simulink model "Vienna_SVM"  (Simulink 7.6)
settings: Solver=ode23tb  StartTime=0.0  StopTime=1.5  RelTol=1e-3
libraries: powerlib x31, powerlib_extras x7, simulink x5
settings Model: Creator=huanglei  LastModifiedBy=huanglei

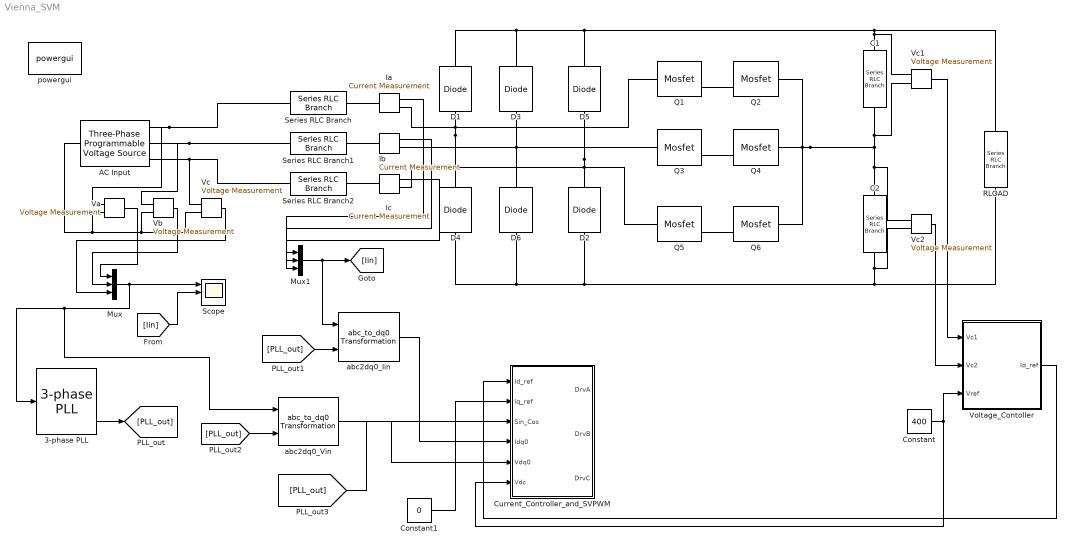
== system Vienna_SVM ==
  3-phase PLL : powerlib_extras/Control  Blocks/3-phase PLL  DialogController=POWERSYS.PowerSysDialog  SystemSampleTime=-1  Par_Init=[0 50]  ParK=[ 180 3200 1 ]  AGC=off
  AC Input : powerlib/Electrical Sources/Three-Phase Programmable Voltage Source  DialogController=POWERSYS.PowerSysDialog  SystemSampleTime=-1  PositiveSequence="[190  0 50]"  VariationEntity=None  VariationType=Step  VariationStep=0.5  VariationRate=10  VariationMagnitude=0.3  VariationFrequency=2  VariationTiming=[1 2]  VariationPhaseA=off  Amplitudes=[1 0.8 1.2 1.0]  TimeValues=[0 0.1 0.15 0.2]  HarmonicGeneration=off  HarmonicA=[3 0.2 -25 0]  HarmonicB=[2 0.15 35 2]  Timing="[0.05  3]"
  C1 : powerlib/Elements/Series RLC Branch  DialogController=POWERSYS.PowerSysDialog  PhysicalDomain=powersysdomain  SubClassName=unknown  LeftPortType=p1  RightPortType=p1  LConnTagsString=__new0  RConnTagsString=__new0  BranchType=C  Resistance=1  Inductance=1e-3  SetiL0=off  InitialCurrent=0  Capacitance=1e-3  Setx0=off  InitialVoltage=0  Measurements=None
  C2 : powerlib/Elements/Series RLC Branch  DialogController=POWERSYS.PowerSysDialog  PhysicalDomain=powersysdomain  SubClassName=unknown  LeftPortType=p1  RightPortType=p1  LConnTagsString=__new0  RConnTagsString=__new0  BranchType=C  Resistance=1  Inductance=1e-3  SetiL0=off  InitialCurrent=0  Capacitance=1e-3  Setx0=off  InitialVoltage=0  Measurements=None
  Constant : Constant  Value=400
  Constant1 : Constant  Value=0
  Current_Controller_and_SVPWM : Subsystem
  D{1..6} (6 alike) : powerlib/Power Electronics/Diode  DialogController=POWERSYS.PowerSysDialog  SystemSampleTime=-1  Ron=0.001  Lon=0  Vf=0.8  IC=0  UseSnubber=off  Rs=500  Cs=250e-9  Measurements=off
  Ia : powerlib/Measurements/Current Measurement  DialogController=POWERSYS.PowerSysDialog  SystemSampleTime=-1  PhasorSimulation=off  OutputType=Complex  PSBequivalent=0
  Ib : powerlib/Measurements/Current Measurement  DialogController=POWERSYS.PowerSysDialog  SystemSampleTime=-1  PhasorSimulation=off  OutputType=Complex  PSBequivalent=0
  Ic : powerlib/Measurements/Current Measurement  DialogController=POWERSYS.PowerSysDialog  SystemSampleTime=-1  PhasorSimulation=off  OutputType=Complex  PSBequivalent=0
  Mux : Mux  Inputs=3
  Mux1 : Mux  Inputs=3
  Q1 : powerlib/Power Electronics/Mosfet  DialogController=POWERSYS.PowerSysDialog  SystemSampleTime=-1  Ron=0.01  Lon=0  Rd=0.01  Vfd=0  IC=0  Rs=1e5  Cs=inf  Measurements=off
  Q{2..6} (5 alike) : powerlib/Power Electronics/Mosfet  DialogController=POWERSYS.PowerSysDialog  SystemSampleTime=-1  Ron=0.1  Lon=0  Rd=0.01  Vfd=0  IC=0  Rs=1e5  Cs=inf  Measurements=off
  RLOAD : powerlib/Elements/Series RLC Branch  DialogController=POWERSYS.PowerSysDialog  PhysicalDomain=powersysdomain  SubClassName=unknown  LeftPortType=p1  RightPortType=p1  LConnTagsString=__new0  RConnTagsString=__new0  BranchType=R  Resistance=80  Inductance=1e-3  SetiL0=off  InitialCurrent=0  Capacitance=1e-6  Setx0=off  InitialVoltage=0  Measurements=None
  Scope : Scope  NumInputPorts=3
      settings: YMin=-5~-5~-5  YMax=5~5~5
  Series RLC Branch : powerlib/Elements/Series RLC Branch  DialogController=POWERSYS.PowerSysDialog  PhysicalDomain=powersysdomain  SubClassName=unknown  LeftPortType=p1  RightPortType=p1  LConnTagsString=__new0  RConnTagsString=__new0  BranchType=RL  Resistance=0  Inductance=3.5e-3  SetiL0=off  InitialCurrent=0  Capacitance=1e-6  Setx0=off  InitialVoltage=0  Measurements=None
  Series RLC Branch1 : powerlib/Elements/Series RLC Branch  DialogController=POWERSYS.PowerSysDialog  PhysicalDomain=powersysdomain  SubClassName=unknown  LeftPortType=p1  RightPortType=p1  LConnTagsString=__new0  RConnTagsString=__new0  BranchType=RL  Resistance=0  Inductance=3.5e-3  SetiL0=off  InitialCurrent=0  Capacitance=1e-6  Setx0=off  InitialVoltage=0  Measurements=None
  Series RLC Branch2 : powerlib/Elements/Series RLC Branch  DialogController=POWERSYS.PowerSysDialog  PhysicalDomain=powersysdomain  SubClassName=unknown  LeftPortType=p1  RightPortType=p1  LConnTagsString=__new0  RConnTagsString=__new0  BranchType=RL  Resistance=0  Inductance=3.5e-3  SetiL0=off  InitialCurrent=0  Capacitance=1e-6  Setx0=off  InitialVoltage=0  Measurements=None
  Va : powerlib/Measurements/Voltage Measurement  DialogController=POWERSYS.PowerSysDialog  SystemSampleTime=-1  PhasorSimulation=off  OutputType=Complex  PSBequivalent=0
  Vb : powerlib/Measurements/Voltage Measurement  DialogController=POWERSYS.PowerSysDialog  SystemSampleTime=-1  PhasorSimulation=off  OutputType=Complex  PSBequivalent=0
  Vc : powerlib/Measurements/Voltage Measurement  DialogController=POWERSYS.PowerSysDialog  SystemSampleTime=-1  PhasorSimulation=off  OutputType=Complex  PSBequivalent=0
  Vc1 : powerlib/Measurements/Voltage Measurement  DialogController=POWERSYS.PowerSysDialog  SystemSampleTime=-1  PhasorSimulation=off  OutputType=Complex  PSBequivalent=0
  Vc2 : powerlib/Measurements/Voltage Measurement  DialogController=POWERSYS.PowerSysDialog  SystemSampleTime=-1  PhasorSimulation=off  OutputType=Complex  PSBequivalent=0
  Voltage_Contoller : Subsystem
  abc2dq0_Iin : powerlib_extras/Measurements/abc_to_dq0 Transformation  DialogController=POWERSYS.PowerSysDialog  SystemSampleTime=-1
  abc2dq0_Vin : powerlib_extras/Measurements/abc_to_dq0 Transformation  DialogController=POWERSYS.PowerSysDialog  SystemSampleTime=-1
  powergui : powerlib/powergui  Priority=1  SystemSampleTime=-1  SimulationMode=Discrete  SampleTime=50e-6  frequency=60  SPID=off  DisableSnubberDevices=off  DisableRonSwitches=off  DisableVfSwitches=off  SwTol=0  Interpol=off  frequencyindice=50  echomessages=off  HookPort=off  DisplayEquations=off  FunctionMessages=off  EnableUseOfTLC=off  x0status=blocks  RestoreLinks=warning  ResistiveCurrentMeasurement=off  Ylog=off  Xlog=on  ShowGrid=off  save=off  variable=ZData  ZoomFFT=off  StartTime=0.0  cycles=1  DisplayStyle=1  FreqAxis=off  MaxFrequency=1000  frequencyindicesteady=1  display=off  methode=off
  wires:
  Vb/1 -> Mux/2
  Va/1 -> Mux/1
  Vc/1 -> Mux/3
  Mux/1 -> Scope/1, 3-phase PLL/1, abc2dq0_Vin/1
  Ia/1 -> Mux1/1
  Ib/1 -> Mux1/2
  Ic/1 -> Mux1/3
  Mux1/1 -> [Iin], abc2dq0_Iin/1
  [Iin] -> Scope/2
  [PLL_out] -> abc2dq0_Iin/2
  3-phase PLL/3 -> [PLL_out]
  [PLL_out] -> abc2dq0_Vin/2
  Constant/1 -> Voltage_Contoller/3(Vref), Current_Controller_and_SVPWM/6(Vdc)
  Vc1/1 -> Voltage_Contoller/1(Vc1)
  Vc2/1 -> Voltage_Contoller/2(Vc2)
  abc2dq0_Iin/1 -> Current_Controller_and_SVPWM/4(Idq0)
  abc2dq0_Vin/1 -> Current_Controller_and_SVPWM/5(Vdq0)
  [PLL_out] -> Current_Controller_and_SVPWM/3(Sin_Cos)
  Constant1/1 -> Current_Controller_and_SVPWM/2(Iq_ref)
  Voltage_Contoller/1(Id_ref) -> Current_Controller_and_SVPWM/1(Id_ref)
  connections:
  AC Input/RConn1 -- Series RLC Branch/LConn1 -- Va/LConn1
  AC Input/RConn2 -- Series RLC Branch1/LConn1 -- Vb/LConn1
  AC Input/RConn3 -- Series RLC Branch2/LConn1 -- Vc/LConn1
  Vc/LConn2 -- Vb/LConn2 -- AC Input/LConn1 -- Va/LConn2
  Series RLC Branch/RConn1 -- Ia/LConn1
  Series RLC Branch1/RConn1 -- Ib/LConn1
  Series RLC Branch2/RConn1 -- Ic/LConn1
  Ia/RConn1 -- D1/LConn1 -- D4/RConn1 -- Q1/RConn1
  D3/LConn1 -- D6/RConn1 -- Ib/RConn1 -- Q3/RConn1
  Ic/RConn1 -- D5/LConn1 -- D2/RConn1 -- Q5/RConn1
  D1/RConn1 -- D3/RConn1 -- D5/RConn1 -- RLOAD/LConn1 -- C1/LConn1 -- Vc1/LConn1
  C2/RConn1 -- D4/LConn1 -- D6/LConn1 -- D2/LConn1 -- RLOAD/RConn1 -- Vc2/LConn2
  Q4/RConn1 -- Q2/RConn1 -- Q6/RConn1 -- C1/RConn1 -- Vc1/LConn2 -- C2/LConn1 -- Vc2/LConn1
  Q1/LConn1 -- Q2/LConn1
  Q3/LConn1 -- Q4/LConn1
  Q5/LConn1 -- Q6/LConn1

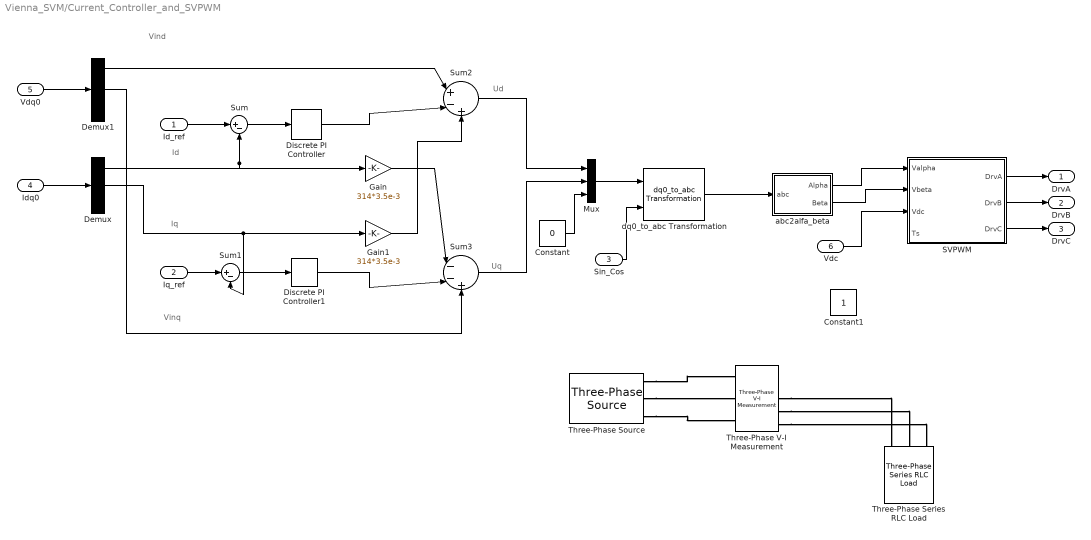
== system Vienna_SVM/Current_Controller_and_SVPWM ==
  note: Ud
  note: Uq
  note: Vind
  note: Vinq
  note: Id
  note: Iq
  Id_ref : Inport
  Iq_ref : Inport  Port=2
  Sin_Cos : Inport  Port=3
  Idq0 : Inport  Port=4
  Vdq0 : Inport  Port=5
  Vdc : Inport  Port=6
  Constant : Constant  Value=0
  Constant1 : Constant
  Demux : Demux  Outputs=3
  Demux1 : Demux  Outputs=3
  Discrete PI Controller : powerlib_extras/Discrete  Control Blocks/Discrete PI Controller  DialogController=POWERSYS.PowerSysDialog  SystemSampleTime=-1  Kp=0.1  Ki=1  Par_Limits=[1e6 -1e6]  Init=0  Ts=50e-6
  Discrete PI Controller1 : powerlib_extras/Discrete  Control Blocks/Discrete PI Controller  DialogController=POWERSYS.PowerSysDialog  SystemSampleTime=-1  Kp=0.1  Ki=1  Par_Limits=[1e6 -1e6]  Init=0  Ts=50e-6
  Gain : Gain  Gain=314*3.5e-3
  Gain1 : Gain  Gain=314*3.5e-3
  Mux : Mux  Inputs=3
  SVPWM : Subsystem
  Sum : Sum  Inputs=|+-
  Sum1 : Sum  Inputs=|+-
  Sum2 : Sum  Inputs=|+-+
  Sum3 : Sum  Inputs=|--+
  Three-Phase Series RLC Load : powerlib/Elements/Three-Phase Series RLC Load  DialogController=POWERSYS.PowerSysDialog  PhysicalDomain=powersysdomain  SubClassName=unknown  LeftPortType=p1  RightPortType=p1  LConnTagsString=A|B|C  Configuration=Y (grounded)  NominalVoltage=1000  NominalFrequency=60  ActivePower=10e3  InductivePower=100  CapacitivePower=100  Measurements=None
  Three-Phase V-I Measurement : powerlib/Measurements/Three-Phase V-I Measurement  DialogController=POWERSYS.PowerSysDialog  SystemSampleTime=-1  VoltageMeasurement=phase-to-ground  SetLabelV=off  LabelV=Vabc  Vpu=off  VpuLL=off  CurrentMeasurement=yes  SetLabelI=off  LabelI=Iabc  Ipu=off  Pbase=100e6  Vbase=500e3  OutputType=Complex  PhasorSimulation=off  PSBequivalent=0
  Three-Phase Source : powerlib/Electrical Sources/Three-Phase Source  DialogController=POWERSYS.PowerSysDialog  SystemSampleTime=-1  Voltage=381  PhaseAngle=0  Frequency=50  InternalConnection=Yn  SpecifyImpedance=on  Resistance=0.8929  Inductance=16.58e-3  ShortCircuitLevel=100e6  BaseVoltage=25e3  XRratio=7
  abc2alfa_beta : Subsystem
  dq0_to_abc Transformation : powerlib_extras/Measurements/dq0_to_abc Transformation  DialogController=POWERSYS.PowerSysDialog  SystemSampleTime=-1
  DrvA : Outport
  DrvB : Outport  Port=2
  DrvC : Outport  Port=3
  wires:
  Id_ref/1 -> Sum/1
  Demux/1 -> Sum/2, Gain/1
  Sum/1 -> Discrete PI Controller/1
  Iq_ref/1 -> Sum1/1
  Sum1/1 -> Discrete PI Controller1/1
  Discrete PI Controller1/1 -> Sum3/2
  Discrete PI Controller/1 -> Sum2/2
  Gain1/1 -> Sum2/3
  Gain/1 -> Sum3/1
  Demux1/1 -> Sum2/1
  Sum2/1 -> Mux/1
  Sum3/1 -> Mux/2
  Constant/1 -> Mux/3
  Mux/1 -> dq0_to_abc Transformation/1
  Sin_Cos/1 -> dq0_to_abc Transformation/2
  Idq0/1 -> Demux/1
  Demux/2 -> Sum1/2, Gain1/1
  Vdq0/1 -> Demux1/1
  Demux1/2 -> Sum3/3
  SVPWM/1(DrvA) -> DrvA/1
  SVPWM/2(DrvB) -> DrvB/1
  SVPWM/3(DrvC) -> DrvC/1
  abc2alfa_beta/1(Alpha) -> SVPWM/1(Valpha)
  abc2alfa_beta/2(Beta) -> SVPWM/2(Vbeta)
  dq0_to_abc Transformation/1 -> abc2alfa_beta/1(abc)
  Vdc/1 -> SVPWM/3(Vdc)
  connections:
  Three-Phase Source/RConn1 -- Three-Phase V-I Measurement/LConn1
  Three-Phase Source/RConn2 -- Three-Phase V-I Measurement/LConn2
  Three-Phase Source/RConn3 -- Three-Phase V-I Measurement/LConn3
  Three-Phase V-I Measurement/RConn3 -- Three-Phase Series RLC Load/LConn3
  Three-Phase V-I Measurement/RConn2 -- Three-Phase Series RLC Load/LConn2
  Three-Phase V-I Measurement/RConn1 -- Three-Phase Series RLC Load/LConn1

== system Vienna_SVM/Voltage_Contoller ==
  Vc1 : Inport
  Vc2 : Inport  Port=2
  Vref : Inport  Port=3
  Discrete PID Controller1 : powerlib_extras/Discrete  Control Blocks/Discrete PID Controller  DialogController=POWERSYS.PowerSysDialog  SystemSampleTime=-1  Kp=1  Ki=1  Kd=1  TcD=1  Par_Limits=[100 -100]  Init=0  Ts=0.5
  Saturation : Saturate
  Sum : Sum  Inputs=|++
  Sum1 : Sum  Inputs=|+-
  Id_ref : Outport
  wires:
  Vc1/1 -> Sum/1
  Vc2/1 -> Sum/2
  Vref/1 -> Sum1/1
  Sum/1 -> Sum1/2
  Sum1/1 -> Discrete PID Controller1/1
  Discrete PID Controller1/1 -> Saturation/1
  Saturation/1 -> Id_ref/1

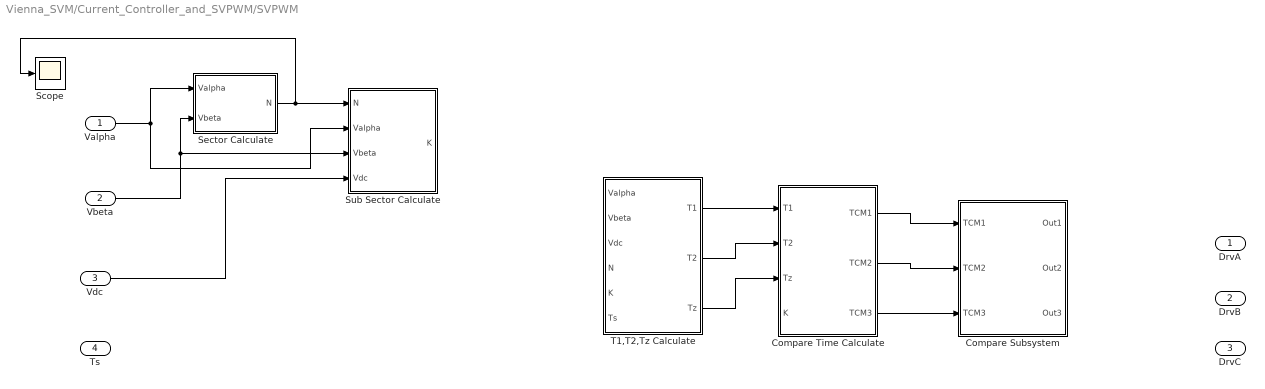
== system Vienna_SVM/Current_Controller_and_SVPWM/SVPWM ==
  Valpha : Inport
  Vbeta : Inport  Port=2
  Vdc : Inport  Port=3
  Ts : Inport  Port=4
  Compare Subsystem : Subsystem
  Compare Time Calculate : Subsystem
  Scope : Scope
  Sector Calculate : Subsystem
  Sub Sector Calculate : Subsystem
  T1,T2,Tz Calculate : Subsystem
  DrvA : Outport
  DrvB : Outport  Port=2
  DrvC : Outport  Port=3
  wires:
  Valpha/1 -> Sector Calculate/1(Valpha), Sub Sector Calculate/2(Valpha)
  Vbeta/1 -> Sector Calculate/2(Vbeta), Sub Sector Calculate/3(Vbeta)
  Sector Calculate/1(N) -> Scope/1, Sub Sector Calculate/1(N)
  Vdc/1 -> Sub Sector Calculate/4(Vdc)
  T1,T2,Tz Calculate/1(T1) -> Compare Time Calculate/1(T1)
  T1,T2,Tz Calculate/2(T2) -> Compare Time Calculate/2(T2)
  T1,T2,Tz Calculate/3(Tz) -> Compare Time Calculate/3(Tz)
  Compare Time Calculate/1(TCM1) -> Compare Subsystem/1(TCM1)
  Compare Time Calculate/3(TCM3) -> Compare Subsystem/3(TCM3)
  Compare Time Calculate/2(TCM2) -> Compare Subsystem/2(TCM2)

== system Vienna_SVM/Current_Controller_and_SVPWM/abc2alfa_beta ==
  abc : Inport
  Demux : Demux  Outputs=3
  Gain : Gain  Gain=2
  Gain1 : Gain  Gain=1/3
  Gain2 : Gain  Gain=sqrt(3)/3
  Scope : Scope  NumInputPorts=3
      settings: YMin=-5~-5~-5  YMax=5~5~5  SaveName=ScopeData2
  Sum : Sum  Inputs=|+--
  Sum2 : Sum  Inputs=|-+
  Alpha : Outport
  Beta : Outport  Port=2
  wires:
  Demux/1 -> Gain/1, Scope/1
  Gain/1 -> Sum/1
  Demux/2 -> Sum/2, Sum2/2, Scope/2
  Demux/3 -> Sum/3, Sum2/1, Scope/3
  Sum/1 -> Gain1/1
  Sum2/1 -> Gain2/1
  abc/1 -> Demux/1
  Gain1/1 -> Alpha/1
  Gain2/1 -> Beta/1

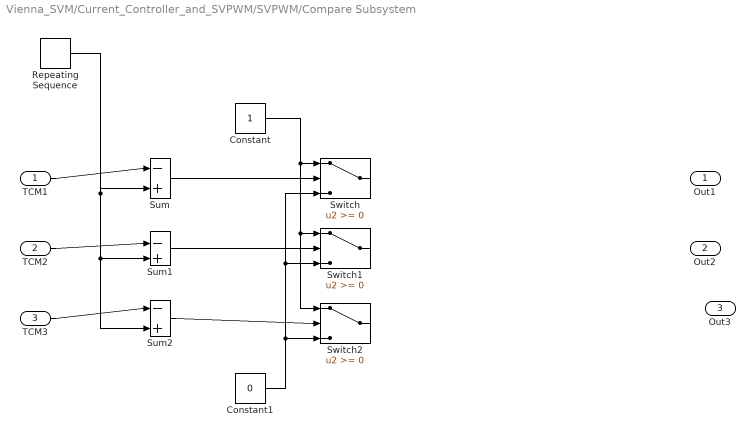
== system Vienna_SVM/Current_Controller_and_SVPWM/SVPWM/Compare Subsystem ==
  TCM1 : Inport
  TCM2 : Inport  Port=2
  TCM3 : Inport  Port=3
  Constant : Constant
  Constant1 : Constant  Value=0
  Repeating Sequence : simulink/Sources/Repeating Sequence  SystemSampleTime=-1  rep_seq_t=[0 1/40000 1/20000]  rep_seq_y=[0 1/40000 0]
  Sum : Sum  Inputs=|-+
  Sum1 : Sum  Inputs=|-+
  Sum2 : Sum  Inputs=|-+
  Switch : Switch
  Switch1 : Switch
  Switch2 : Switch
  Out1 : Outport
  Out2 : Outport  Port=2
  Out3 : Outport  Port=3
  wires:
  TCM1/1 -> Sum/1
  TCM2/1 -> Sum1/1
  TCM3/1 -> Sum2/1
  Repeating Sequence/1 -> Sum2/2, Sum1/2, Sum/2
  Sum1/1 -> Switch1/2
  Sum/1 -> Switch/2
  Sum2/1 -> Switch2/2
  Constant/1 -> Switch2/1, Switch1/1, Switch/1
  Constant1/1 -> Switch/3, Switch1/3, Switch2/3

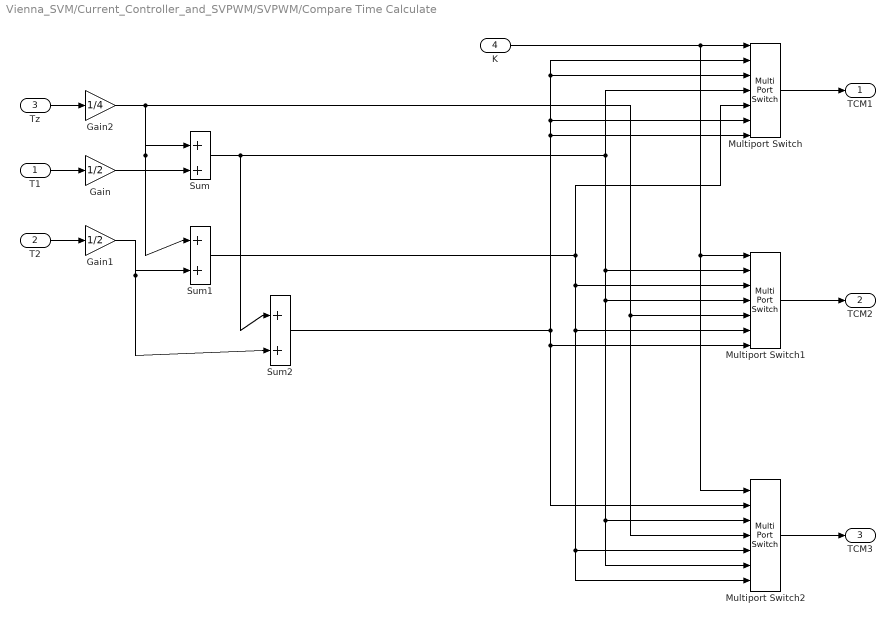
== system Vienna_SVM/Current_Controller_and_SVPWM/SVPWM/Compare Time Calculate ==
  T1 : Inport
  T2 : Inport  Port=2
  Tz : Inport  Port=3
  K : Inport  Port=4
  Gain : Gain  Gain=1/2
  Gain1 : Gain  Gain=1/2
  Gain2 : Gain  Gain=1/4
  Multiport Switch : MultiPortSwitch  Inputs=6  zeroidx=off
  Multiport Switch1 : MultiPortSwitch  Inputs=6  zeroidx=off
  Multiport Switch2 : MultiPortSwitch  Inputs=6  zeroidx=off
  Sum : Sum  Inputs=|++
  Sum1 : Sum  Inputs=|++
  Sum2 : Sum  Inputs=|++
  TCM1 : Outport
  TCM2 : Outport  Port=2
  TCM3 : Outport  Port=3
  wires:
  T1/1 -> Gain/1
  T2/1 -> Gain1/1
  Tz/1 -> Gain2/1
  Gain2/1 -> Sum/1, Sum1/1, Multiport Switch2/4, Multiport Switch1/5
  Gain/1 -> Sum/2
  Gain1/1 -> Sum1/2, Sum2/2
  Sum/1 -> Sum2/1, Multiport Switch1/2, Multiport Switch1/4, Multiport Switch2/6, Multiport Switch2/3, Multiport Switch/4
  K/1 -> Multiport Switch/1, Multiport Switch2/1, Multiport Switch1/1
  Sum1/1 -> Multiport Switch2/7, Multiport Switch2/5, Multiport Switch1/6, Multiport Switch1/3, Multiport Switch/5
  Sum2/1 -> Multiport Switch/2, Multiport Switch/3, Multiport Switch/6, Multiport Switch/7, Multiport Switch2/2, Multiport Switch1/7
  Multiport Switch/1 -> TCM1/1
  Multiport Switch1/1 -> TCM2/1
  Multiport Switch2/1 -> TCM3/1

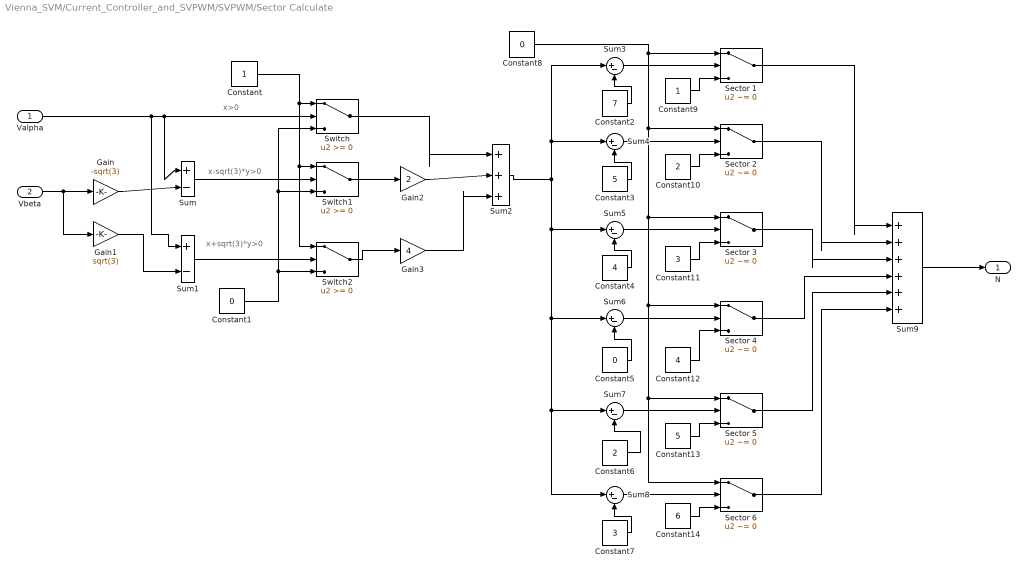
== system Vienna_SVM/Current_Controller_and_SVPWM/SVPWM/Sector Calculate ==
  note: x>0
  note: x-sqrt(3)*y>0
  note: x+sqrt(3)*y>0
  Valpha : Inport
  Vbeta : Inport  Port=2
  Constant : Constant
  Constant1 : Constant  Value=0
  Constant10 : Constant  Value=2
  Constant11 : Constant  Value=3
  Constant12 : Constant  Value=4
  Constant13 : Constant  Value=5
  Constant14 : Constant  Value=6
  Constant2 : Constant  Value=7
  Constant3 : Constant  Value=5
  Constant4 : Constant  Value=4
  Constant5 : Constant  Value=0
  Constant6 : Constant  Value=2
  Constant7 : Constant  Value=3
  Constant8 : Constant  Value=0
  Constant9 : Constant
  Gain : Gain  Gain=-sqrt(3)
  Gain1 : Gain  Gain=sqrt(3)
  Gain2 : Gain  Gain=2
  Gain3 : Gain  Gain=4
  Sector {1..6} (6 alike) : Switch  Criteria=u2 ~= 0
  Sum{,1,3..8} (8 alike) : Sum  Inputs=|+-
  Sum2 : Sum  Inputs=|+++
  Sum9 : Sum  Inputs=|++++++
  Switch : Switch
  Switch1 : Switch
  Switch2 : Switch
  N : Outport
  wires:
  Valpha/1 -> Switch/2, Sum/1, Sum1/1
  Vbeta/1 -> Gain/1, Gain1/1
  Gain/1 -> Sum/2
  Gain1/1 -> Sum1/2
  Sum/1 -> Switch1/2
  Sum1/1 -> Switch2/2
  Constant/1 -> Switch/1, Switch2/1, Switch1/1
  Constant1/1 -> Switch/3, Switch1/3, Switch2/3
  Switch1/1 -> Gain2/1
  Switch2/1 -> Gain3/1
  Gain2/1 -> Sum2/2
  Switch/1 -> Sum2/1
  Gain3/1 -> Sum2/3
  Constant2/1 -> Sum3/2
  Constant3/1 -> Sum4/2
  Constant4/1 -> Sum5/2
  Constant5/1 -> Sum6/2
  Constant6/1 -> Sum7/2
  Constant7/1 -> Sum8/2
  Sum2/1 -> Sum3/1, Sum4/1, Sum5/1, Sum6/1, Sum8/1, Sum7/1
  Sum3/1 -> Sector 1/2
  Sum4/1 -> Sector 2/2
  Sum5/1 -> Sector 3/2
  Sum6/1 -> Sector 4/2
  Sum7/1 -> Sector 5/2
  Sum8/1 -> Sector 6/2
  Constant8/1 -> Sector 1/1, Sector 2/1, Sector 3/1, Sector 4/1, Sector 6/1, Sector 5/1
  Constant9/1 -> Sector 1/3
  Constant10/1 -> Sector 2/3
  Constant11/1 -> Sector 3/3
  Constant12/1 -> Sector 4/3
  Constant13/1 -> Sector 5/3
  Constant14/1 -> Sector 6/3
  Sector 1/1 -> Sum9/1
  Sector 2/1 -> Sum9/2
  Sector 3/1 -> Sum9/3
  Sector 6/1 -> Sum9/6
  Sector 5/1 -> Sum9/5
  Sector 4/1 -> Sum9/4
  Sum9/1 -> N/1

== system Vienna_SVM/Current_Controller_and_SVPWM/SVPWM/Sub Sector Calculate ==
  N : Inport
  Valpha : Inport  Port=2
  Vbeta : Inport  Port=3
  Vdc : Inport  Port=4
  2-level Sector Calculate : Subsystem
  Constant : Constant  Value=3
  Divide : Product  Inputs=*/
  Rotate to Sector 1 : Subsystem
  Sum : Sum  Inputs=|-+
  K : Outport
  wires:
  Valpha/1 -> Rotate to Sector 1/1(alpha)
  N/1 -> Rotate to Sector 1/3(N)
  Vbeta/1 -> Rotate to Sector 1/2(Beta)
  Vdc/1 -> Divide/1
  Constant/1 -> Divide/2
  Rotate to Sector 1/1(alpha_R) -> Sum/2
  Divide/1 -> Sum/1
  Sum/1 -> 2-level Sector Calculate/1(alpha)
  Rotate to Sector 1/2(beta_R) -> 2-level Sector Calculate/2(bata)
  2-level Sector Calculate/1(K) -> K/1

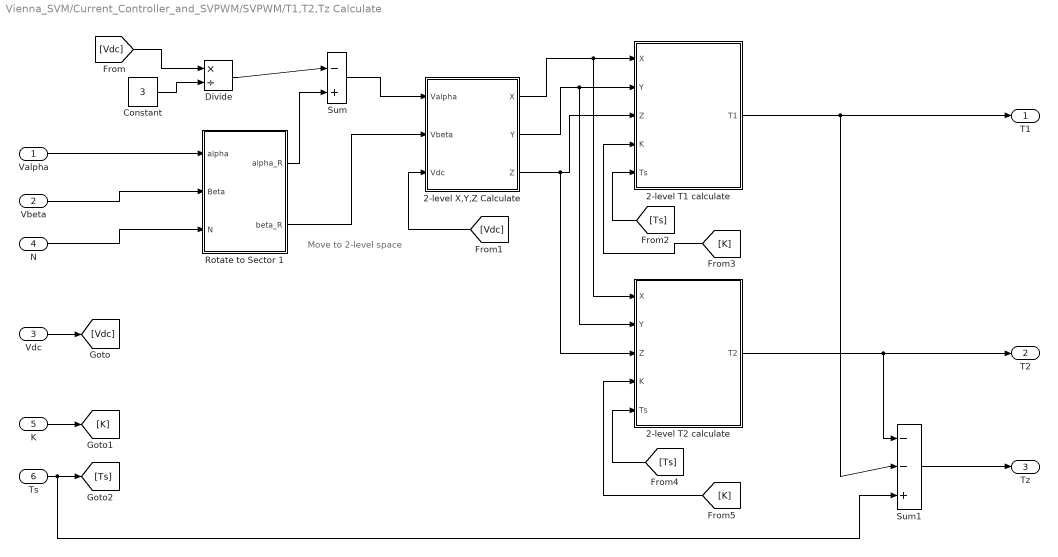
== system Vienna_SVM/Current_Controller_and_SVPWM/SVPWM/T1,T2,Tz Calculate ==
  note: Move to 2-level space
  Valpha : Inport
  Vbeta : Inport  Port=2
  Vdc : Inport  Port=3
  N : Inport  Port=4
  K : Inport  Port=5
  Ts : Inport  Port=6
  2-level T1 calculate : Subsystem
  2-level T2 calculate : Subsystem
  2-level X,Y,Z Calculate : Subsystem
  Constant : Constant  Value=3
  Divide : Product  Inputs=*/
  Rotate to Sector 1 : Subsystem
  Sum : Sum  Inputs=|-+
  Sum1 : Sum  Inputs=|--+
  T1 : Outport
  T2 : Outport  Port=2
  Tz : Outport  Port=3
  wires:
  Valpha/1 -> Rotate to Sector 1/1(alpha)
  Vbeta/1 -> Rotate to Sector 1/2(Beta)
  N/1 -> Rotate to Sector 1/3(N)
  Vdc/1 -> [Vdc]
  Constant/1 -> Divide/2
  [Vdc] -> Divide/1
  Divide/1 -> Sum/1
  Rotate to Sector 1/1(alpha_R) -> Sum/2
  [Vdc] -> 2-level X,Y,Z Calculate/3(Vdc)
  2-level X,Y,Z Calculate/1(X) -> 2-level T1 calculate/1(X), 2-level T2 calculate/1(X)
  2-level X,Y,Z Calculate/2(Y) -> 2-level T1 calculate/2(Y), 2-level T2 calculate/2(Y)
  2-level X,Y,Z Calculate/3(Z) -> 2-level T1 calculate/3(Z), 2-level T2 calculate/3(Z)
  K/1 -> [K]
  Ts/1 -> [Ts], Sum1/3
  Sum/1 -> 2-level X,Y,Z Calculate/1(Valpha)
  Rotate to Sector 1/2(beta_R) -> 2-level X,Y,Z Calculate/2(Vbeta)
  [Ts] -> 2-level T1 calculate/5(Ts)
  [K] -> 2-level T1 calculate/4(K)
  [Ts] -> 2-level T2 calculate/5(Ts)
  [K] -> 2-level T2 calculate/4(K)
  2-level T1 calculate/1(T1) -> T1/1, Sum1/2
  2-level T2 calculate/1(T2) -> T2/1, Sum1/1
  Sum1/1 -> Tz/1

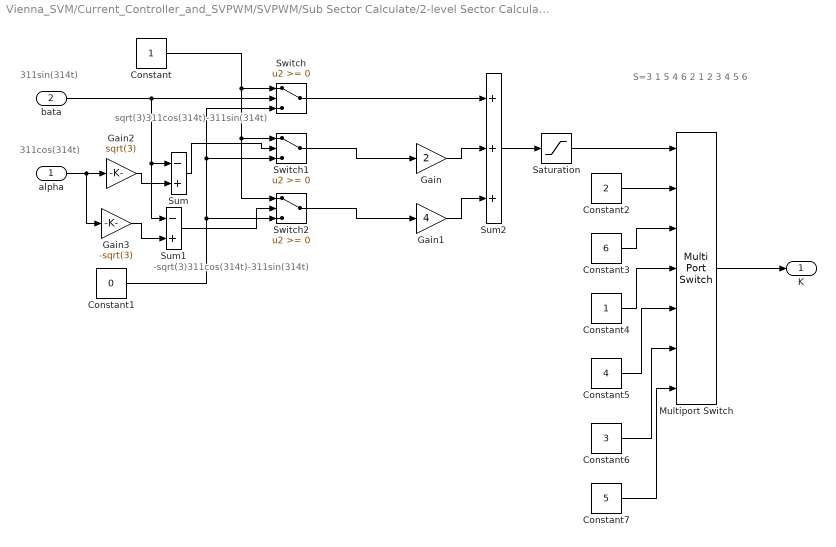
== system Vienna_SVM/Current_Controller_and_SVPWM/SVPWM/Sub Sector Calculate/2-level Sector Calculate ==
  note: 311sin(314t)
  note: 311cos(314t)
  note: sqrt(3)311cos(314t)-311sin(314t)
  note: -sqrt(3)311cos(314t)-311sin(314t)
  note: S=3    1    5    4    6    2
      |
      |      1    2    3    4    5    6
  alpha : Inport
  bata : Inport  Port=2
  Constant : Constant
  Constant1 : Constant  Value=0
  Constant2 : Constant  Value=2
  Constant3 : Constant  Value=6
  Constant4 : Constant
  Constant5 : Constant  Value=4
  Constant6 : Constant  Value=3
  Constant7 : Constant  Value=5
  Gain : Gain  Gain=2  SaturateOnIntegerOverflow=on  OutDataTypeStr=Inherit: Same as input  ParamDataTypeStr=Inherit: Same as input
  Gain1 : Gain  Gain=4  SaturateOnIntegerOverflow=on  OutDataTypeStr=Inherit: Same as input  ParamDataTypeStr=Inherit: Same as input
  Gain2 : Gain  Gain=sqrt(3)  SaturateOnIntegerOverflow=on  OutDataTypeStr=Inherit: Same as input  ParamDataTypeStr=Inherit: Same as input
  Gain3 : Gain  Gain=-sqrt(3)  SaturateOnIntegerOverflow=on  OutDataTypeStr=Inherit: Same as input  ParamDataTypeStr=Inherit: Same as input
  Multiport Switch : MultiPortSwitch  Inputs=6  zeroidx=off
  Saturation : Saturate  UpperLimit=6  LowerLimit=1
  Sum : Sum  Inputs=-+  SaturateOnIntegerOverflow=on
  Sum1 : Sum  Inputs=-+  SaturateOnIntegerOverflow=on
  Sum2 : Sum  Inputs=+++  SaturateOnIntegerOverflow=on
  Switch : Switch  SaturateOnIntegerOverflow=on
  Switch1 : Switch  SaturateOnIntegerOverflow=on
  Switch2 : Switch  SaturateOnIntegerOverflow=on
  K : Outport
  wires:
  Constant/1 -> Switch/1, Switch1/1, Switch2/1
  bata/1 -> Sum/1, Sum1/1, Switch/2
  Constant1/1 -> Switch/3, Switch1/3, Switch2/3
  alpha/1 -> Gain2/1, Gain3/1
  Gain2/1 -> Sum/2
  Gain3/1 -> Sum1/2
  Sum/1 -> Switch1/2
  Sum1/1 -> Switch2/2
  Switch1/1 -> Gain/1
  Switch/1 -> Sum2/1
  Gain/1 -> Sum2/2
  Gain1/1 -> Sum2/3
  Switch2/1 -> Gain1/1
  Sum2/1 -> Saturation/1
  Saturation/1 -> Multiport Switch/1
  Constant2/1 -> Multiport Switch/2
  Constant3/1 -> Multiport Switch/3
  Constant4/1 -> Multiport Switch/4
  Constant5/1 -> Multiport Switch/5
  Constant6/1 -> Multiport Switch/6
  Constant7/1 -> Multiport Switch/7
  Multiport Switch/1 -> K/1

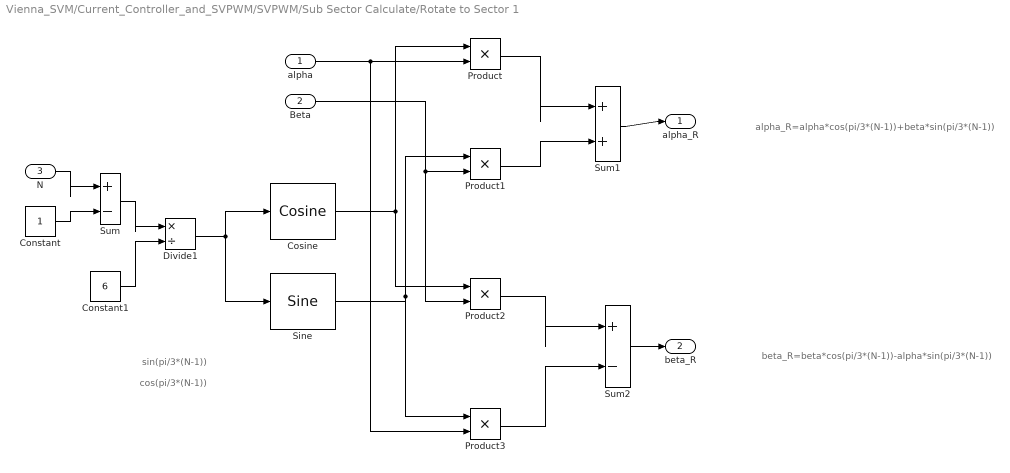
== system Vienna_SVM/Current_Controller_and_SVPWM/SVPWM/Sub Sector Calculate/Rotate to Sector 1 ==
  note: sin(pi/3*(N-1))
  note: cos(pi/3*(N-1))
  note: alpha_R=alpha*cos(pi/3*(N-1))+beta*sin(pi/3*(N-1))
  note: beta_R=beta*cos(pi/3*(N-1))-alpha*sin(pi/3*(N-1))
  alpha : Inport
  Beta : Inport  Port=2
  N : Inport  Port=3
  Constant : Constant
  Constant1 : Constant  Value=6
  Cosine : simulink/Lookup Tables/Cosine  SystemSampleTime=-1  Formula=cos(2*pi*u)  NumDataPoints=(2^5)+1  OutputWordLength=16
  Divide1 : Product  Inputs=*/
  Product{,1..3} (4 alike) : Product  RndMeth=Zero
  Sine : simulink/Lookup Tables/Sine  SystemSampleTime=-1  Formula=sin(2*pi*u)  NumDataPoints=(2^5)+1  OutputWordLength=16
  Sum : Sum  Inputs=|+-
  Sum1 : Sum  Inputs=|++
  Sum2 : Sum  Inputs=|+-
  alpha_R : Outport
  beta_R : Outport  Port=2
  wires:
  N/1 -> Sum/1
  Constant/1 -> Sum/2
  Constant1/1 -> Divide1/2
  Sum/1 -> Divide1/1
  Divide1/1 -> Cosine/1, Sine/1
  Cosine/1 -> Product/1, Product2/1
  Sine/1 -> Product1/1, Product3/1
  alpha/1 -> Product/2, Product3/2
  Beta/1 -> Product1/2, Product2/2
  Product2/1 -> Sum2/1
  Product3/1 -> Sum2/2
  Product/1 -> Sum1/1
  Product1/1 -> Sum1/2
  Sum1/1 -> alpha_R/1
  Sum2/1 -> beta_R/1

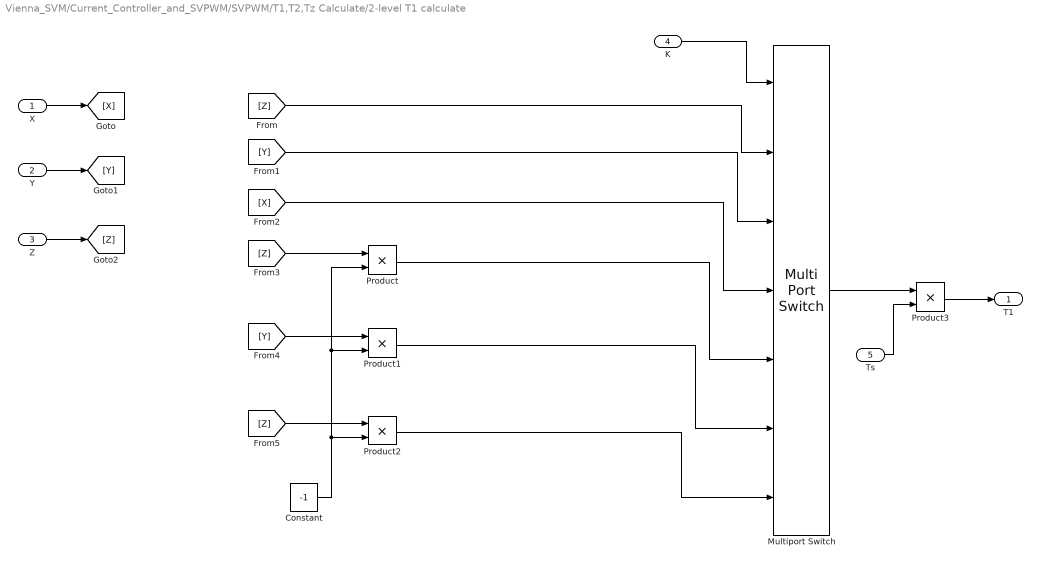
== system Vienna_SVM/Current_Controller_and_SVPWM/SVPWM/T1,T2,Tz Calculate/2-level T1 calculate ==
  X : Inport
  Y : Inport  Port=2
  Z : Inport  Port=3
  K : Inport  Port=4
  Ts : Inport  Port=5
  Constant : Constant  Value=-1
  Multiport Switch : MultiPortSwitch  Inputs=6  zeroidx=off
  Product{,1..3} (4 alike) : Product  RndMeth=Zero
  T1 : Outport
  wires:
  K/1 -> Multiport Switch/1
  X/1 -> [X]
  Y/1 -> [Y]
  Z/1 -> [Z]
  [Z] -> Multiport Switch/2
  [Y] -> Multiport Switch/3
  [X] -> Multiport Switch/4
  [Z] -> Product/1
  Product/1 -> Multiport Switch/5
  [Y] -> Product1/1
  Product1/1 -> Multiport Switch/6
  [Z] -> Product2/1
  Product2/1 -> Multiport Switch/7
  Constant/1 -> Product/2, Product1/2, Product2/2
  Multiport Switch/1 -> Product3/1
  Ts/1 -> Product3/2
  Product3/1 -> T1/1

== system Vienna_SVM/Current_Controller_and_SVPWM/SVPWM/T1,T2,Tz Calculate/2-level T2 calculate ==
  X : Inport
  Y : Inport  Port=2
  Z : Inport  Port=3
  K : Inport  Port=4
  Ts : Inport  Port=5
  Constant : Constant  Value=-1
  Multiport Switch : MultiPortSwitch  Inputs=6  zeroidx=off
  Product{,1..3} (4 alike) : Product  RndMeth=Zero
  T2 : Outport
  wires:
  K/1 -> Multiport Switch/1
  X/1 -> Multiport Switch/2, Product/1
  Product/1 -> Multiport Switch/5
  Z/1 -> Multiport Switch/6, Product2/1
  Y/1 -> Multiport Switch/7, Product1/1
  Product1/1 -> Multiport Switch/4
  Product2/1 -> Multiport Switch/3
  Constant/1 -> Product2/2, Product1/2, Product/2
  Multiport Switch/1 -> Product3/1
  Ts/1 -> Product3/2
  Product3/1 -> T2/1

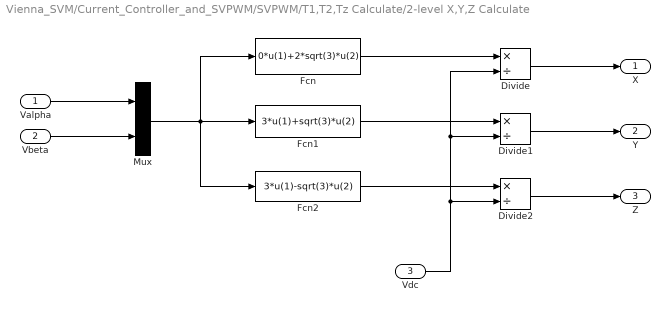
== system Vienna_SVM/Current_Controller_and_SVPWM/SVPWM/T1,T2,Tz Calculate/2-level X,Y,Z Calculate ==
  Valpha : Inport
  Vbeta : Inport  Port=2
  Vdc : Inport  Port=3
  Divide : Product  Inputs=*/
  Divide1 : Product  Inputs=*/
  Divide2 : Product  Inputs=*/
  Fcn : Fcn  Expr=0*u(1)+2*sqrt(3)*u(2)
  Fcn1 : Fcn  Expr=3*u(1)+sqrt(3)*u(2)
  Fcn2 : Fcn  Expr=3*u(1)-sqrt(3)*u(2)
  Mux : Mux  Inputs=2
  X : Outport
  Y : Outport  Port=2
  Z : Outport  Port=3
  wires:
  Valpha/1 -> Mux/1
  Vbeta/1 -> Mux/2
  Fcn/1 -> Divide/1
  Fcn1/1 -> Divide1/1
  Fcn2/1 -> Divide2/1
  Vdc/1 -> Divide/2, Divide1/2, Divide2/2
  Divide/1 -> X/1
  Divide1/1 -> Y/1
  Divide2/1 -> Z/1
  Mux/1 -> Fcn1/1, Fcn/1, Fcn2/1

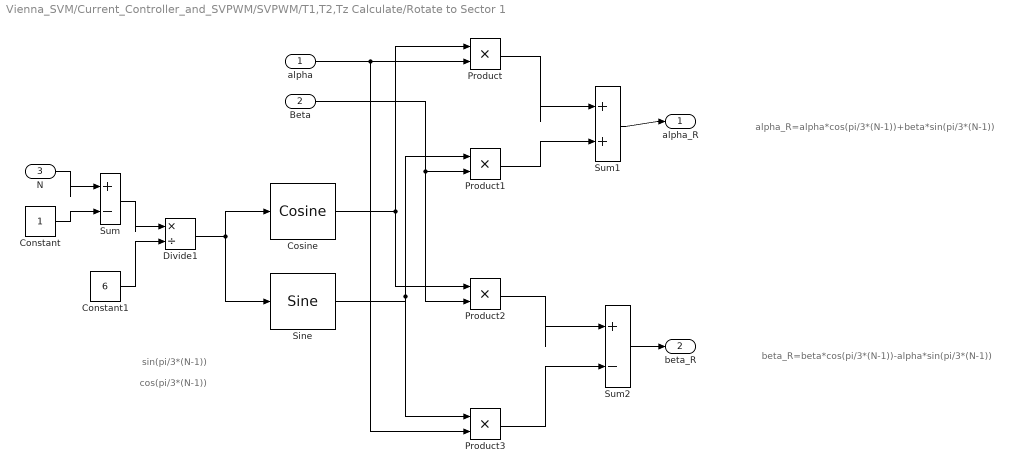
== system Vienna_SVM/Current_Controller_and_SVPWM/SVPWM/T1,T2,Tz Calculate/Rotate to Sector 1 ==
  note: sin(pi/3*(N-1))
  note: cos(pi/3*(N-1))
  note: alpha_R=alpha*cos(pi/3*(N-1))+beta*sin(pi/3*(N-1))
  note: beta_R=beta*cos(pi/3*(N-1))-alpha*sin(pi/3*(N-1))
  alpha : Inport
  Beta : Inport  Port=2
  N : Inport  Port=3
  Constant : Constant
  Constant1 : Constant  Value=6
  Cosine : simulink/Lookup Tables/Cosine  SystemSampleTime=-1  Formula=cos(2*pi*u)  NumDataPoints=(2^5)+1  OutputWordLength=16
  Divide1 : Product  Inputs=*/
  Product{,1..3} (4 alike) : Product  RndMeth=Zero
  Sine : simulink/Lookup Tables/Sine  SystemSampleTime=-1  Formula=sin(2*pi*u)  NumDataPoints=(2^5)+1  OutputWordLength=16
  Sum : Sum  Inputs=|+-
  Sum1 : Sum  Inputs=|++
  Sum2 : Sum  Inputs=|+-
  alpha_R : Outport
  beta_R : Outport  Port=2
  wires:
  N/1 -> Sum/1
  Constant/1 -> Sum/2
  Constant1/1 -> Divide1/2
  Sum/1 -> Divide1/1
  Divide1/1 -> Cosine/1, Sine/1
  Cosine/1 -> Product/1, Product2/1
  Sine/1 -> Product1/1, Product3/1
  alpha/1 -> Product/2, Product3/2
  Beta/1 -> Product1/2, Product2/2
  Product2/1 -> Sum2/1
  Product3/1 -> Sum2/2
  Product/1 -> Sum1/1
  Product1/1 -> Sum1/2
  Sum1/1 -> alpha_R/1
  Sum2/1 -> beta_R/1
